simulink model "sldemo_mrv_nonlinear_controller"  (Simulink 7.6)
settings: Solver=FixedStepDiscrete  StartTime=0.0  StopTime=10.0  RelTol=1e-3
settings Model: Creator=The MathWorks Inc.
settings OptimizationCC: InlineParams=on
settings RTWCC: ProcessScript=grt_make_rtw_hook

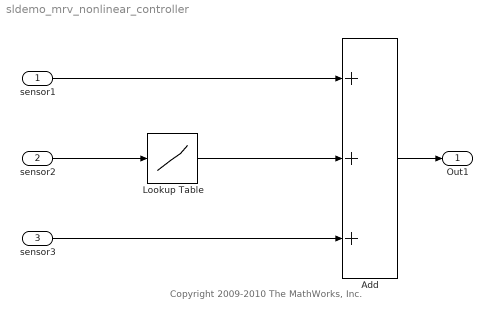
== system sldemo_mrv_nonlinear_controller ==
  note: Copyright 2009-2010 The MathWorks, Inc.
  sensor1 : Inport
  sensor2 : Inport  Port=2
  sensor3 : Inport  Port=3
  Add : Sum  Inputs=+++  SampleTime=.01
  Lookup Table : Lookup  InputValues=[-5:5]  Table=tanh([-5:5])
  Out1 : Outport
  wires:
  sensor2/1 -> Lookup Table/1
  Lookup Table/1 -> Add/2
  sensor3/1 -> Add/3
  sensor1/1 -> Add/1
  Add/1 -> Out1/1
